simulink model "lab_5_rlc_sim"  (R2024a)
settings: Solver=FixedStepAuto  StartTime=0.0  StopTime=0.1  FixedStep=dt  RelTol=1e-3
values from neighbouring files (symbols this model uses):
  den = [R*L*C L R]    [lab_5_task_1.m]    (also in lab_5_task_2.m)
  dt = 1/1e6    (= 1e-06)    [lab_5_task_1.m]    (also in lab_5_task_2.m)
  num = [L 0]    [lab_5_task_1.m]    (also in lab_5_task_2.m)
settings Model: Creator=Jakub  LastModifiedBy=jakubsz
settings RTWCC: GPUComputeCapability=3.5

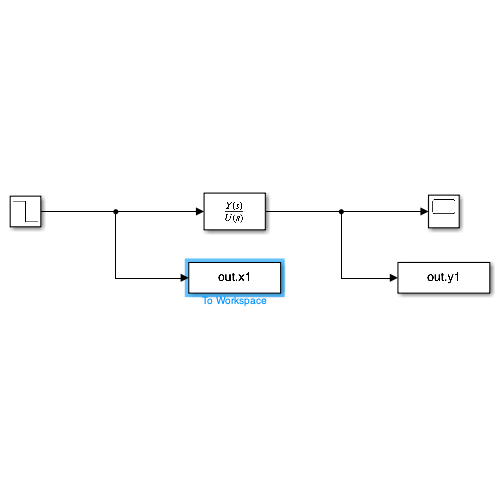
[thumbnail: Simulink's stored preview of the top-level diagram]
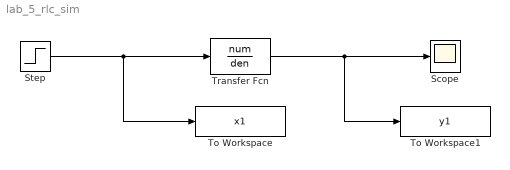
== system lab_5_rlc_sim ==
  Scope : Scope
  Step : Step  Time=dt  Before=1  After=0  SampleTime=0
  To Workspace : ToWorkspace  VariableName=x1  SampleTime=-1
  To Workspace1 : ToWorkspace  VariableName=y1  SampleTime=-1
  Transfer Fcn : TransferFcn  Numerator=num  Denominator=den
  wires:
  Transfer Fcn/1 -> To Workspace1/1, Scope/1
  Step/1 -> To Workspace/1, Transfer Fcn/1
